simulink model "c6713dskwdnoisf"  (Simulink 6.0)
settings: Solver=FixedStepDiscrete  StartTime=0.0  StopTime=inf  RelTol=1e-3
PreLoadFcn:
  | load dspwlets;
undefined symbols (not defined in the file or in its folder): bit, lod
libraries: dspsigattribs x8, c6713dsklib x2, dspmlti3 x2, dspsigops x2, c6000tgtpreflib x1
settings Model: RequirementInfo=9  CovMetricSettings=d  Creator=don  LastModifiedBy=thartley  ExtModeTrigMode=oneshot  ExtModeArmWhenConnect=off  ProdHWDeviceType=TI C6000
settings DataIOCC: LimitDataPoints=off  SaveOutput=off  SaveTime=off  SignalLoggingName=sigsOut
settings OptimizationCC: BlockReduction=off  BooleanDataType=off  InlineParams=on  RollThreshold=2
settings DebuggingCC: CheckExecutionContextPreStartOutputMsg=on  CheckExecutionContextRuntimeOutputMsg=on  SolverPrmCheckMsg=none  IntegerOverflowMsg=none
settings HardwareCC: ProdBitPerLong=40  ProdEndianess=LittleEndian  ProdHWDeviceType=TI C6000
settings ModelReferenceCC: UpdateModelReferenceTargets=IfOutOfDate
settings RTWCC: SystemTargetFile=ti_c6000.tlc  TemplateMakefile=ti_c6000.tmf  ProcessScript=ti_c6000_make_rtw_hook
settings CodeAppCC: PrefixModelToSubsysFcnNames=off
settings STFCustomTargetCC: TargetFcnLib=ansi_tfl_tmw.mat  MatFileLogging=on  LifeSpan=inf  SystemTargetFile=ti_c6000.tlc  ActivateCallback=c6000_callback('ActivateCallback',hSrc,hDlg);
settings GRTTargetCC: ModelReferenceCompliant=off  LifeSpan=inf
settings CustomProperty: DataType=RTWOptions_EnumType_S__A_matlab_toolbox_rtw_targets_tic6000_tic6000_ti_c6000_BoardType  Value=C6713DSK
settings EnumStrPairs: String=C6416DSK
settings SFSimCC: SFSimApplyToAllLibs=on  SFSimBuildMode=Incremental

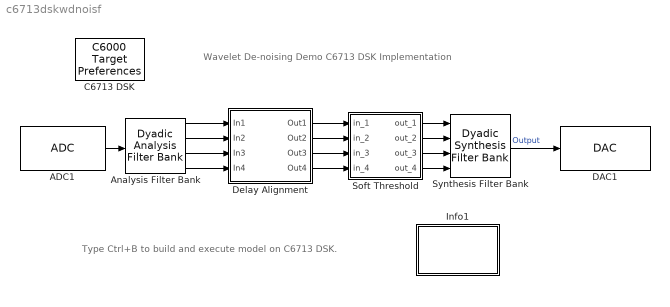
== system c6713dskwdnoisf ==
  note: Wavelet De-noising Demo
      | C6713 DSK Implementation
  note: Type Ctrl+B to build
      | and execute model
      | on C6713 DSK.
  ADC1 : c6713dsklib/ADC  ADCsource=Mic In  MicGain=off  Stereo=off  SampleRate=44.1 kHz  CodecDataFormat=16-bit  OutputDataType=Double  Scaling=Normalize  SourceGain=0.0  FrameSize=64
  Analysis Filter Bank : dspmlti3/Dyadic Analysis Filter Bank  hl=lod  hh=hid  numLevels=3  tree=Asymmetric
  C6713 DSK : c6000tgtpreflib/C6000 Target Preferences
  DAC1 : c6713dsklib/DAC  CodecDataFormat=16-bit  Scaling=Normalize  DacAtten=0.0  OverflowMode=Wrap
  Delay Alignment : Subsystem
  Info1 : Subsystem
      mask Type: Frame-Based Simulation Info
      mask Display: disp('Info')
  Soft Threshold : Subsystem  mask(Soft Threshold){st=[3 2 1 0]}
      mask prompts: st "Vector of thresholds for each level:"
      mask help: Apply a soft threshold (deadzone transfer function) to each signal in the decomposition. First threshold applies to top-most filter bank output.
      mask init:
      | x=([-1 1 NaN 0 0 NaN -1 -.5 .5 1]+1)/2*.7+.15;
      | y=([0 0 NaN -1 1 NaN -1 0 0 1]+1)/2*.7+.05;
      mask Help: Vector of thresholds for each decomposition level.
      mask Display:
      | text(.1,.9,'Dead Zone')
      | plot(x,y)
  Synthesis Filter Bank : dspmlti3/Dyadic Synthesis Filter Bank  hl=lor  hh=hir  numLevels=3  tree=Asymmetric
  wires:
  ADC1/1 -> Analysis Filter Bank/1
  Analysis Filter Bank/4 -> Delay Alignment/4(In4)
  Analysis Filter Bank/3 -> Delay Alignment/3(In3)
  Analysis Filter Bank/2 -> Delay Alignment/2(In2)
  Analysis Filter Bank/1 -> Delay Alignment/1(In1)
  Delay Alignment/4(Out4) -> Soft Threshold/4(in_4)
  Delay Alignment/3(Out3) -> Soft Threshold/3(in_3)
  Delay Alignment/2(Out2) -> Soft Threshold/2(in_2)
  Delay Alignment/1(Out1) -> Soft Threshold/1(in_1)
  Soft Threshold/1(out_1) -> Synthesis Filter Bank/1
  Soft Threshold/2(out_2) -> Synthesis Filter Bank/2
  Soft Threshold/3(out_3) -> Synthesis Filter Bank/3
  Soft Threshold/4(out_4) -> Synthesis Filter Bank/4
  Synthesis Filter Bank/1 -> DAC1/1  "Output"

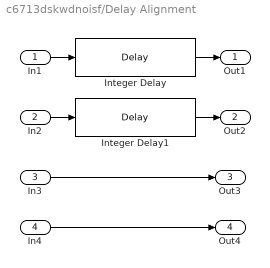
== system c6713dskwdnoisf/Delay Alignment ==
  In1 : Inport
  In2 : Inport  Port=2
  In3 : Inport  Port=3
  In4 : Inport  Port=4
  Integer Delay : dspsigops/Delay  dly_unit=Samples  delay=3*(length(lod)-1)  ic_detail=off  dif_ic_for_ch=off  dif_ic_for_dly=off  ic=0  reset_popup=None
  Integer Delay1 : dspsigops/Delay  dly_unit=Samples  delay=length(lod) - 1  ic_detail=off  dif_ic_for_ch=off  dif_ic_for_dly=off  ic=0  reset_popup=None
  Out1 : Outport
  Out2 : Outport  Port=2
  Out3 : Outport  Port=3
  Out4 : Outport  Port=4
  wires:
  In3/1 -> Out3/1
  In4/1 -> Out4/1
  In2/1 -> Integer Delay1/1
  Integer Delay1/1 -> Out2/1
  In1/1 -> Integer Delay/1
  Integer Delay/1 -> Out1/1

== system c6713dskwdnoisf/Info1 ==
  note: Demonstration of wavelet de-noising
      |
      | Set the threshold levels in the "Soft Threshold" block
      | to alter the de-noising characteristics of the system:
      |
      | Threshold=[0 0 0 0]  -> No de-noising
      | (perfect reconstruction)
      |
      | Threshold=[3 2 1 0] -> Moderate de-noising
      | (removes small-scale content from signal)

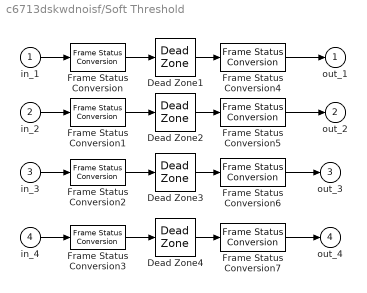
== system c6713dskwdnoisf/Soft Threshold ==
  in_1 : Inport
  in_2 : Inport  Port=2
  in_3 : Inport  Port=3
  in_4 : Inport  Port=4
  Dead Zone1 : DeadZone  LowerValue=-st(1)  UpperValue=st(1)  ZeroCross=off  SaturateOnIntegerOverflow=on
  Dead Zone2 : DeadZone  LowerValue=-st(2)  UpperValue=st(2)  ZeroCross=off  SaturateOnIntegerOverflow=on
  Dead Zone3 : DeadZone  LowerValue=-st(3)  UpperValue=st(3)  ZeroCross=off  SaturateOnIntegerOverflow=on
  Dead Zone4 : DeadZone  LowerValue=-st(4)  UpperValue=st(4)  ZeroCross=off  SaturateOnIntegerOverflow=on
  Frame Status Conversion{,1..3} (4 alike) : dspsigattribs/Frame Status Conversion  growRefPort=off  outframe=Sample-based
  Frame Status Conversion{4..7} (4 alike) : dspsigattribs/Frame Status Conversion  growRefPort=off  outframe=Frame-based
  out_1 : Outport  InitialOutput=0
  out_2 : Outport  Port=2  InitialOutput=0
  out_3 : Outport  Port=3  InitialOutput=0
  out_4 : Outport  Port=4  InitialOutput=0
  wires:
  in_1/1 -> Frame Status Conversion/1
  Frame Status Conversion/1 -> Dead Zone1/1
  in_2/1 -> Frame Status Conversion1/1
  Frame Status Conversion1/1 -> Dead Zone2/1
  in_3/1 -> Frame Status Conversion2/1
  Frame Status Conversion2/1 -> Dead Zone3/1
  in_4/1 -> Frame Status Conversion3/1
  Frame Status Conversion3/1 -> Dead Zone4/1
  Dead Zone1/1 -> Frame Status Conversion4/1
  Frame Status Conversion4/1 -> out_1/1
  Dead Zone2/1 -> Frame Status Conversion5/1
  Frame Status Conversion5/1 -> out_2/1
  Dead Zone3/1 -> Frame Status Conversion6/1
  Frame Status Conversion6/1 -> out_3/1
  Dead Zone4/1 -> Frame Status Conversion7/1
  Frame Status Conversion7/1 -> out_4/1
